simulink model "fmcomms5"  (R2019b)
settings: Solver=ode45  StartTime=0.0  StopTime=Inf  RelTol=1e-3  EnableMultiTasking=on
undefined symbols (not defined in the file): ad9361
libraries: simulink x4, dspsrcs4 x2
settings Model: Creator=ACozma  LastModifiedBy=bhisma
settings DataIOCC: LimitDataPoints=on  SaveFormat=Array  ReturnWorkspaceOutputs=off
settings OptimizationCC: LifeSpan=inf
settings DebuggingCC: UnderspecifiedInitializationDetection=Classic  MergeDetectMultiDrivingBlocksExec=none  SolverPrmCheckMsg=warning  SFUnexpectedBacktrackingDiag=warning  SFNoUnconditionalDefaultTransitionDiag=warning  SFExecutionAtInitializationDiag=none  ArithmeticOperatorsInVariantConditions=warning
settings HardwareCC: ProdBitPerPointer=32  ProdBitPerSizeT=32  ProdBitPerPtrDiffT=32  ProdLargestAtomicFloat=None  ProdIntDivRoundTo=Undefined  ProdEndianess=Unspecified  ProdWordSize=32  ProdHWDeviceType=32-bit Generic
settings ModelReferenceCC: PropagateSignalLabelsOutOfModel=off
settings SFSimCC: SimUseLocalCustomCode=off  CustomCodeUndefinedFunction=UseInterfaceOnly
settings RTWCC: RTWUseLocalCustomCode=off
settings CodeAppCC: StateflowObjectComments=on
settings GRTTargetCC: TargetLangStandard=C89/C90 (ANSI)  GeneratePreprocessorConditionals=Disable all
settings ConfigComp: CovMetricSettings=dw  CovHtmlReporting=on  CovSaveCumulativeToWorkspaceVar=on  CovSaveSingleToWorkspaceVar=on  CovExternalEMLEnable=off  CovSFcnEnable=off

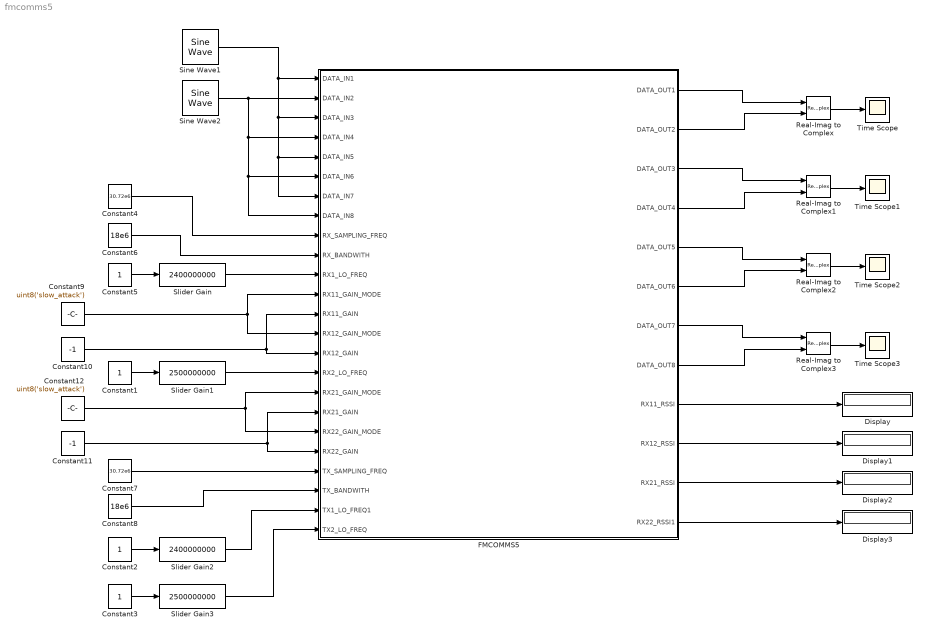
== system fmcomms5 ==
  Constant{1..3,5} (4 alike) : Constant  SampleTime=-1
  Constant10 : Constant  Value=-1  SampleTime=-1
  Constant11 : Constant  Value=-1  SampleTime=-1
  Constant12 : Constant  Value=uint8('slow_attack')  SampleTime=-1
  Constant4 : Constant  Value=30.72e6  SampleTime=-1
  Constant6 : Constant  Value=18e6  SampleTime=-1
  Constant7 : Constant  Value=30.72e6  SampleTime=-1
  Constant8 : Constant  Value=18e6  SampleTime=-1
  Constant9 : Constant  Value=uint8('slow_attack')  SampleTime=-1
  Display{,1..3} (4 alike) : Display
  FMCOMMS5 : Subsystem
  Real-Imag to Complex{,1..3} (4 alike) : RealImagToComplex
  Sine Wave1 : dspsrcs4/Sine Wave  Amplitude=32768  Frequency=100  Phase=0  SampleMode=Discrete  OutComplex=Real  CompMethod=Trigonometric fcn  TableSize=Speed  SampleTime=1/10000  SamplesPerFrame=32768  ResetState=Catch up to simulation time  OutputFrames=on  dataType=double  wordLen=16  udDataType=sfix(16)  fracBitsMode=Best precision  numFracBits=15  OutDataTypeStr=double  LastOutDataTypeStr=double
  Sine Wave2 : dspsrcs4/Sine Wave  Amplitude=32768  Frequency=100  Phase=pi/2  SampleMode=Discrete  OutComplex=Real  CompMethod=Trigonometric fcn  TableSize=Speed  SampleTime=1/10000  SamplesPerFrame=32768  ResetState=Catch up to simulation time  OutputFrames=on  dataType=double  wordLen=16  udDataType=sfix(16)  fracBitsMode=Best precision  numFracBits=15  OutDataTypeStr=double  LastOutDataTypeStr=double
  Slider Gain : simulink/Math Operations/Slider Gain  gain=2400000000  low=200000  high=6000000000
  Slider Gain1 : simulink/Math Operations/Slider Gain  gain=2500000000  low=200000  high=6000000000
  Slider Gain2 : simulink/Math Operations/Slider Gain  gain=2400000000  low=200000  high=6000000000
  Slider Gain3 : simulink/Math Operations/Slider Gain  gain=2500000000  low=200000  high=6000000000
  Time Scope{,1..3} (4 alike) : Scope
  wires:
  Sine Wave1/1 -> FMCOMMS5/7(DATA_IN7), FMCOMMS5/5(DATA_IN5), FMCOMMS5/3(DATA_IN3), FMCOMMS5/1(DATA_IN1)
  Sine Wave2/1 -> FMCOMMS5/6(DATA_IN6), FMCOMMS5/8(DATA_IN8), FMCOMMS5/4(DATA_IN4), FMCOMMS5/2(DATA_IN2)
  Constant5/1 -> Slider Gain/1
  Slider Gain/1 -> FMCOMMS5/11(RX1_LO_FREQ)
  Constant1/1 -> Slider Gain1/1
  Slider Gain1/1 -> FMCOMMS5/16(RX2_LO_FREQ)
  Constant2/1 -> Slider Gain2/1
  Slider Gain2/1 -> FMCOMMS5/23(TX1_LO_FREQ1)
  Constant3/1 -> Slider Gain3/1
  Slider Gain3/1 -> FMCOMMS5/24(TX2_LO_FREQ)
  Constant4/1 -> FMCOMMS5/9(RX_SAMPLING_FREQ)
  Constant6/1 -> FMCOMMS5/10(RX_BANDWITH)
  Constant7/1 -> FMCOMMS5/21(TX_SAMPLING_FREQ)
  Constant8/1 -> FMCOMMS5/22(TX_BANDWITH)
  Constant9/1 -> FMCOMMS5/12(RX11_GAIN_MODE), FMCOMMS5/14(RX12_GAIN_MODE)
  Constant10/1 -> FMCOMMS5/15(RX12_GAIN), FMCOMMS5/13(RX11_GAIN)
  Constant12/1 -> FMCOMMS5/19(RX22_GAIN_MODE), FMCOMMS5/17(RX21_GAIN_MODE)
  Constant11/1 -> FMCOMMS5/18(RX21_GAIN), FMCOMMS5/20(RX22_GAIN)
  FMCOMMS5/1(DATA_OUT1) -> Real-Imag to Complex/1
  Real-Imag to Complex/1 -> Time Scope/1
  FMCOMMS5/2(DATA_OUT2) -> Real-Imag to Complex/2
  FMCOMMS5/3(DATA_OUT3) -> Real-Imag to Complex1/1
  Real-Imag to Complex1/1 -> Time Scope1/1
  FMCOMMS5/4(DATA_OUT4) -> Real-Imag to Complex1/2
  FMCOMMS5/5(DATA_OUT5) -> Real-Imag to Complex2/1
  Real-Imag to Complex2/1 -> Time Scope2/1
  FMCOMMS5/6(DATA_OUT6) -> Real-Imag to Complex2/2
  FMCOMMS5/7(DATA_OUT7) -> Real-Imag to Complex3/1
  Real-Imag to Complex3/1 -> Time Scope3/1
  FMCOMMS5/8(DATA_OUT8) -> Real-Imag to Complex3/2
  FMCOMMS5/9(RX11_RSSI) -> Display/1
  FMCOMMS5/10(RX12_RSSI) -> Display1/1
  FMCOMMS5/11(RX21_RSSI) -> Display2/1
  FMCOMMS5/12(RX22_RSSI1) -> Display3/1

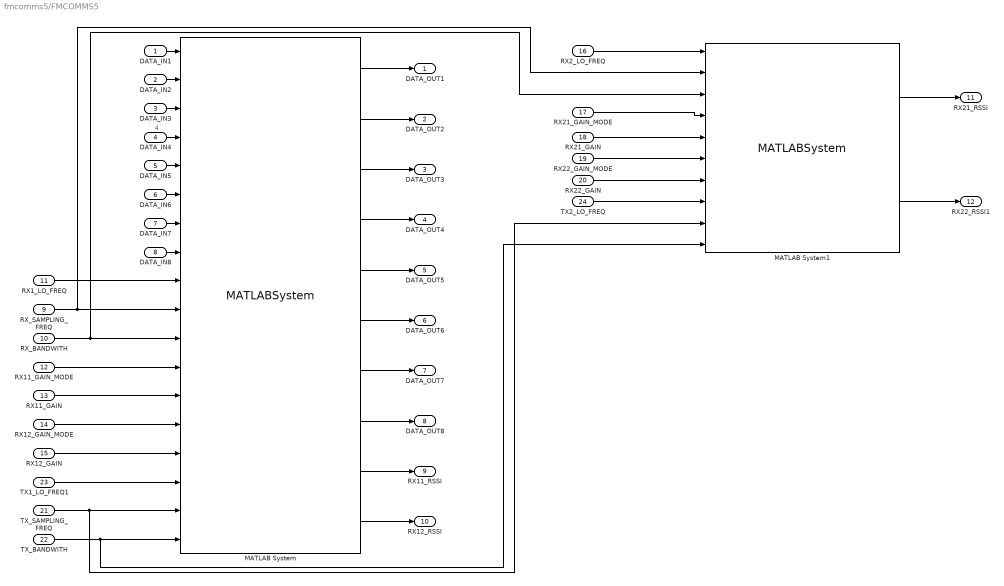
== system fmcomms5/FMCOMMS5 ==
  note: 4
  DATA_IN1 : Inport
  DATA_IN2 : Inport  Port=2
  DATA_IN3 : Inport  Port=3
  DATA_IN4 : Inport  Port=4
  DATA_IN5 : Inport  Port=5
  DATA_IN6 : Inport  Port=6
  DATA_IN7 : Inport  Port=7
  DATA_IN8 : Inport  Port=8
  RX_SAMPLING_FREQ : Inport  Port=9
  RX_BANDWITH : Inport  Port=10
  RX1_LO_FREQ : Inport  Port=11
  RX11_GAIN_MODE : Inport  Port=12
  RX11_GAIN : Inport  Port=13
  RX12_GAIN_MODE : Inport  Port=14
  RX12_GAIN : Inport  Port=15
  RX2_LO_FREQ : Inport  Port=16
  RX21_GAIN_MODE : Inport  Port=17
  RX21_GAIN : Inport  Port=18
  RX22_GAIN_MODE : Inport  Port=19
  RX22_GAIN : Inport  Port=20
  TX_SAMPLING_FREQ : Inport  Port=21
  TX_BANDWITH : Inport  Port=22
  TX1_LO_FREQ1 : Inport  Port=23
  TX2_LO_FREQ : Inport  Port=24
  MATLAB System : MATLABSystem  DialogController=sysobjdialog.BlockDynDialog  System=iio_sys_obj  SimulateUsing=Interpreted execution  ip_address=10.50.1.121  dev_name=ad9361-1  in_ch_no=8  in_ch_size=32768  out_ch_no=8  out_ch_size=8192
      mask Type: iio_sys_obj
      mask Display:
      | disp('ad9361-1');
      | port_label('input',1,'DATA_IN1');
      | port_label('input',2,'DATA_IN2');
      | port_label('input',3,'DATA_IN3');
      | port_label('input',4,'DATA_IN4');
      | port_label('input',5,'DATA_IN5');
      | port_label('input',6,'DATA_IN6');
      | port_label('input',7,'DATA_IN7');
      | port_label('input',8,'DATA_IN8');
      | port_label('input',9,'RX_LO_FREQ');
      | port_label('input',10,'RX_SAMPLING_FREQ');
      | port_label('input',11,'RX_RF_BANDWIDTH');
      | port_label('input',12,'RX1_GAIN_MODE');
      | port_label('input',13,'RX1_GAIN');
      | port_label('input',14,'RX2_GAIN_MODE');
      | port_label('input',15,'RX2_GAIN');
      | port_label('input',16,'TX_LO_FREQ');
      | port_label('input',17,'TX_SAMPLING_FREQ');
      | port_label('input',18,'TX_RF_BANDWIDTH');
      | port_label('output',1,'DATA_OUT1');
      | port_label('output',2,'DATA_OUT2');
      | port_label('output',3,'DATA_OUT3');
      | port_label('output',4,'DATA_OUT4');
      | port_label('output',5,'DATA_OUT5');
      | port_label('output',6,'DATA_OUT6');
      | port_label('output',7,'DATA_OUT7');
      | port_label('output',8,'DATA_OUT8');
      | port_label('output',9,'RX1_RSSI');
      | port_label('output',10,'RX2_RSSI');
  MATLAB System1 : MATLABSystem  DialogController=sysobjdialog.BlockDynDialog  System=iio_sys_obj  SimulateUsing=Interpreted execution  ip_address=10.50.1.121  dev_name=ad9361-2  in_ch_no=0  in_ch_size=32768  out_ch_no=0  out_ch_size=8192
      mask Type: iio_sys_obj
      mask Display:
      | disp('ad9361-2');
      | port_label('input',1,'RX_LO_FREQ');
      | port_label('input',2,'RX_SAMPLING_FREQ');
      | port_label('input',3,'RX_RF_BANDWIDTH');
      | port_label('input',4,'RX1_GAIN_MODE');
      | port_label('input',5,'RX1_GAIN');
      | port_label('input',6,'RX2_GAIN_MODE');
      | port_label('input',7,'RX2_GAIN');
      | port_label('input',8,'TX_LO_FREQ');
      | port_label('input',9,'TX_SAMPLING_FREQ');
      | port_label('input',10,'TX_RF_BANDWIDTH');
      | port_label('output',1,'RX1_RSSI');
      | port_label('output',2,'RX2_RSSI');
  DATA_OUT1 : Outport
  DATA_OUT2 : Outport  Port=2
  DATA_OUT3 : Outport  Port=3
  DATA_OUT4 : Outport  Port=4
  DATA_OUT5 : Outport  Port=5
  DATA_OUT6 : Outport  Port=6
  DATA_OUT7 : Outport  Port=7
  DATA_OUT8 : Outport  Port=8
  RX11_RSSI : Outport  Port=9
  RX12_RSSI : Outport  Port=10
  RX21_RSSI : Outport  Port=11
  RX22_RSSI1 : Outport  Port=12
  wires:
  MATLAB System/7 -> DATA_OUT7/1
  MATLAB System/1 -> DATA_OUT1/1
  MATLAB System/8 -> DATA_OUT8/1
  MATLAB System/2 -> DATA_OUT2/1
  RX22_GAIN/1 -> MATLAB System1/7
  TX_SAMPLING_FREQ/1 -> MATLAB System1/9, MATLAB System/17
  TX_BANDWITH/1 -> MATLAB System1/10, MATLAB System/18
  RX_BANDWITH/1 -> MATLAB System1/3, MATLAB System/11
  RX11_GAIN_MODE/1 -> MATLAB System/12
  MATLAB System/5 -> DATA_OUT5/1
  MATLAB System/6 -> DATA_OUT6/1
  RX22_GAIN_MODE/1 -> MATLAB System1/6
  RX_SAMPLING_FREQ/1 -> MATLAB System1/2, MATLAB System/10
  MATLAB System/10 -> RX12_RSSI/1
  MATLAB System/9 -> RX11_RSSI/1
  MATLAB System/3 -> DATA_OUT3/1
  MATLAB System/4 -> DATA_OUT4/1
  RX12_GAIN/1 -> MATLAB System/15
  RX21_GAIN/1 -> MATLAB System1/5
  RX11_GAIN/1 -> MATLAB System/13
  RX21_GAIN_MODE/1 -> MATLAB System1/4
  RX12_GAIN_MODE/1 -> MATLAB System/14
  TX2_LO_FREQ/1 -> MATLAB System1/8
  RX2_LO_FREQ/1 -> MATLAB System1/1
  TX1_LO_FREQ1/1 -> MATLAB System/16
  RX1_LO_FREQ/1 -> MATLAB System/9
  DATA_IN8/1 -> MATLAB System/8
  DATA_IN7/1 -> MATLAB System/7
  DATA_IN6/1 -> MATLAB System/6
  DATA_IN5/1 -> MATLAB System/5
  DATA_IN4/1 -> MATLAB System/4
  DATA_IN3/1 -> MATLAB System/3
  DATA_IN2/1 -> MATLAB System/2
  DATA_IN1/1 -> MATLAB System/1
  MATLAB System1/1 -> RX21_RSSI/1
  MATLAB System1/2 -> RX22_RSSI1/1
